simulink model "truck_turn_pid"  (R2024a)
settings: Solver=VariableStepAuto  StartTime=0.0  StopTime=1000  RelTol=1e-3
libraries: slpidlib x2, truck_lib x2
settings Model: Creator=adriaeik  LastModifiedBy=eikel

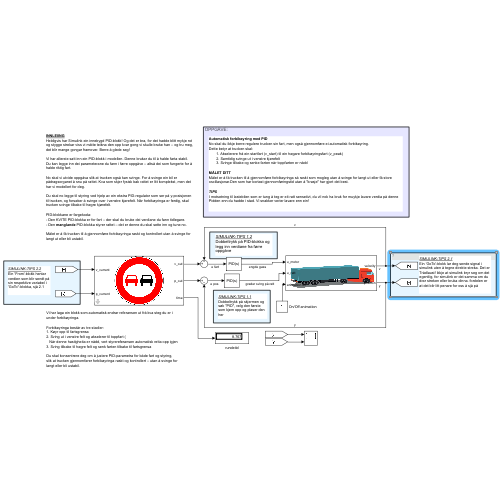
[thumbnail: Simulink's stored preview of the top-level diagram]
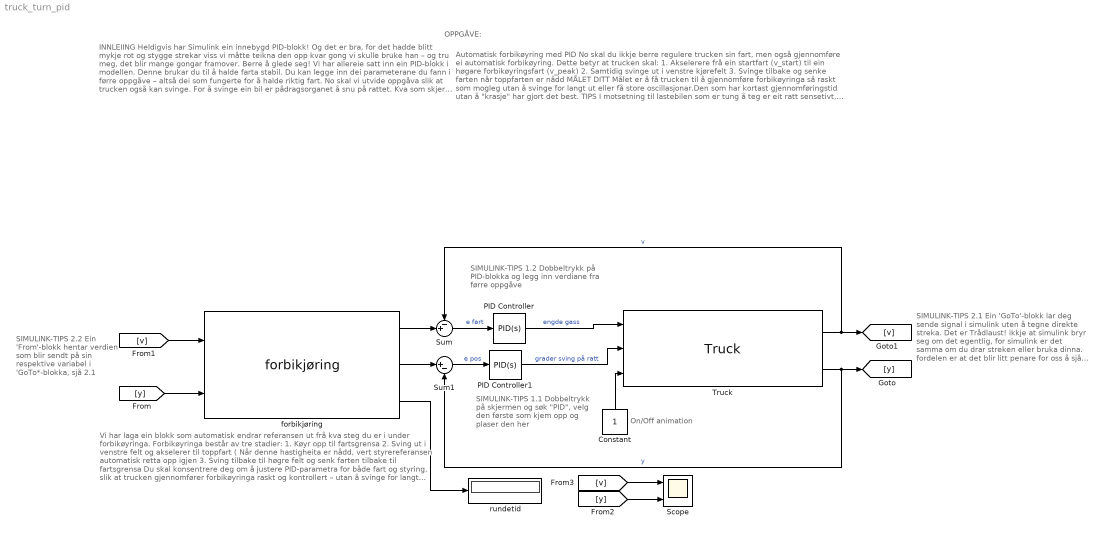
== system truck_turn_pid ==
  note: SIMULINK-TIPS 1.2
      | Dobbeltrykk på PID-blokka og legg inn verdiane fra førre oppgåve
  note: On/Off animation
  note: SIMULINK-TIPS 1.1
      | Dobbeltrykk på skjermen og søk "PID", velg den første som kjem opp og plaser den her
  note: SIMULINK-TIPS 2.1
      | Ein 'GoTo'-blokk lar deg sende signal i simulink uten å tegne direkte streka. Det er Trådlaust! ikkje at simulink bryr seg om det egentlig, for simulink er det samma om du drar streken eller bruka dinna. fordelen er at det blir litt penare for oss å sjå på
  note: INNLEIING
      | Heldigvis har Simulink ein innebygd PID-blokk! Og det er bra, for det hadde blitt mykje rot og stygge strekar viss vi måtte teikna den opp kvar gong vi skulle bruke han – og tru meg, det blir mange gongar framover. Berre å glede seg!
      |
      | Vi har allereie satt inn ein PID-blokk i modellen. Denne brukar du til å halde farta stabil. Du kan legge inn dei parameterane du fann i førre oppgåve – altså dei som fungerte for å halde riktig fart.
      |
      | No skal vi utvide oppgåva slik at trucken også kan svinge. For å svinge ein bil er pådragsorganet å snu på rattet. Kva som skjer fysisk bak rattet er litt komplekst, men det har vi modellert for deg.
      |
      | Du skal no legge til styring ved hjelp av ein ekstra PID-regulator som ser på y-posisjonen til trucken, og forsøker å svinge over i venstre kjørefelt. Når forbikøyringa er ferdig, skal trucken svinge tilbake til høgre kjørefelt.
      |
      | PID-blokkane er fargekoda:
      | - Den KVITE PID-blokka er for fart – der skal du bruke dei verdiane du fann tidlegare.
      | - Den manglande PID-blokka styrer rattet – det er denne du skal sette inn og tune no.
      |
      | Målet er å få trucken til å gjennomføre forbikøyringa raskt og kontrollert utan å svinge for langt ut eller bli ustabil.
  note: OPPGÅVE:
  note: Vi har laga ein blokk som automatisk endrar referansen ut frå kva steg du er i under forbikøyringa.
      |
      | Forbikøyringa består av tre stadier:
      | 1. Køyr opp til fartsgrensa
      | 2. Sving ut i venstre felt og akselerer til toppfart (
      | Når denne hastigheita er nådd, vert styrereferansen automatisk retta opp igjen
      | 3. Sving tilbake til høgre felt og senk farten tilbake til fartsgrensa
      |
      | Du skal konsentrere deg om å justere PID-parametra for både fart og styring,
      | slik at trucken gjennomfører forbikøyringa raskt og kontrollert – utan å svinge for langt eller bli ustabil.
  note: Automatisk forbikøyring med PID
      | No skal du ikkje berre regulere trucken sin fart, men også gjennomføre ei automatisk forbikøyring.
      | Dette betyr at trucken skal:
      | 1. Akselerere frå ein startfart (v_start) til ein høgare forbikøyringsfart (v_peak)
      | 2. Samtidig svinge ut i venstre kjørefelt
      | 3. Svinge tilbake og senke farten når toppfarten er nådd
      |
      | MÅLET DITT
      | Målet er å få trucken til å gjennomføre forbikøyringa så raskt som mogleg utan å svinge for langt ut eller få store oscillasjonar.Den som har kortast gjennomføringstid utan å "krasje" har gjort det best.
      |
      | TIPS
      | I motsetning til lastebilen som er tung å teg er eit ratt sensetivt, du vil nok ha bruk for muykje lavare verdia på denne Pidden enn du hadde i stad. Vi snakker verier lavare enn ein!
  note: SIMULINK-TIPS 2.2
      | Ein 'From'-blokk hentar verdien som blir sendt på sin respektive variabel i 'GoTo*-blokka, sjå 2.1
  Constant : Constant
  PID Controller : slpidlib/PID Controller  Controller=PID  Form=Parallel  TimeDomain=Continuous-time  UseExternalTs=off  SampleTime=-1  IntegratorMethod=Forward Euler  FilterMethod=Forward Euler  ControllerParametersSource=internal  P=1500000  I=9  UseKiTs=off  D=100  UseExternalDerivativeSource=off  N=100  UseFilter=on  TunerSelectOption=Transfer Function Based (PID Tuner App)  InitialConditionSource=internal  InitialConditionForIntegrator=0  InitialConditionForFilter=0  DifferentiatorICPrevScaledInput=0  ExternalReset=none  TrackingMode=off  Kt=1  LimitOutput=off  SatLimitsSource=internal  UpperSaturationLimit=inf  LowerSaturationLimit=-inf  LinearizeAsGain=on  AntiWindupMode=none  Kb=1  LimitIntegrator=off  UpperIntegratorSaturationLimit=inf  LowerIntegratorSaturationLimit=-inf  POutMin=[]  POutMax=[]  IOutMin=[]  IOutMax=[]  DOutMin=[]  DOutMax=[]  NOutMin=[]  NOutMax=[]  SumOutMin=[]  SumOutMax=[]  SaturationOutMin=[]  SaturationOutMax=[]  PParamMin=[]  PParamMax=[]  IParamMin=[]  IParamMax=[]  DParamMin=[]  DParamMax=[]  NParamMin=[]  NParamMax=[]  KbParamMin=[]  KbParamMax=[]  KtParamMin=[]  KtParamMax=[]  KbOutMin=[]  KbOutMax=[]  KtOutMin=[]  KtOutMax=[]  IntegratorOutMin=[]  IntegratorOutMax=[]  FilterOutMin=[]  FilterOutMax=[]  SumI1OutMin=[]  SumI1OutMax=[]  SumI2OutMin=[]  SumI2OutMax=[]  SumI3OutMin=[]  SumI3OutMax=[]  SumI4OutMin=[]  SumI4OutMax=[]  SumDOutMin=[]  SumDOutMax=[]  DifferentiatorOutMin=[]  DifferentiatorOutMax=[]  FilterDiffOutCoefMin=[]  FilterDiffOutCoefMax=[]  ReciprocalOutMin=[]  ReciprocalOutMax=[]  SumDenOutMin=[]  SumDenOutMax=[]  SumNumOutMin=[]  SumNumOutMax=[]  DivideOutMin=[]  DivideOutMax=[]  UdiffTsProdOutMin=[]  UdiffTsProdOutMax=[]  NTsProdOutMin=[]  NTsProdOutMax=[]  UintegralTsProdOutMin=[]  UintegralTsProdOutMax=[]  UngainTsProdOutMin=[]  UngainTsProdOutMax=[]  ClampingZeroOutDataTypeStr=Inherit: Inherit via back propagation  ClampingZeroOutMin=[]  ClampingZeroOutMax=[]  FilterDenConstantOutDataTypeStr=Inherit: Inherit via back propagation  FilterDenConstantOutMin=[]  FilterDenConstantOutMax=[]  PCopyOutDataTypeStr=Inherit: Inherit via back propagation  PCopyOutMin=[]  PCopyOutMax=[]  NCopyOutDataTypeStr=Inherit: Inherit via back propagation  NCopyOutMin=[]  NCopyOutMax=[]  IntegratorContinuousStateAttributes=''  IntegratorStateMustResolveToSignalObject=off  IntegratorRTWStateStorageClass=Auto  FilterContinuousStateAttributes=''  FilterStateMustResolveToSignalObject=off  FilterRTWStateStorageClass=Auto  ParallelPVariant=InternalParameters  IdealPVariant=Disabled  IVariant=InternalParameters  DVariant=InternalParameters  IntegratorVariant=Continuous  SatVariant=Disabled  AWVariant=Passthrough  PCopyVariant=Disabled  TRVariant=Disabled  FdbkBlocksVariant=Forward  IdealPFdbkVariant=Disabled  SatFdbkVariant=Disabled  DerivativeFilterVariant=ContFilter  NVariant=InternalParameters  NCopyVariant=Disabled  FilterICVariant=InternalICsFilter  IntegratorICVariant=InternalICs  ExternalResetVariant=Disabled  TRSumVariant=Passthrough  SumFdbkVariant=Disabled  SumVariant=Sum_PID  TsampFilterVariant=InternalTs  TsampNgainVariant=Passthrough  TsampIntegralVariant=Disabled_SignalSpec  ExternalSaturationOutDataTypeStr=Inherit: Same as second input  DerivativeSourceVariant=ErrorSignal
  PID Controller1 : slpidlib/PID Controller  Controller=PID  Form=Parallel  TimeDomain=Continuous-time  UseExternalTs=off  SampleTime=-1  IntegratorMethod=Forward Euler  FilterMethod=Forward Euler  ControllerParametersSource=internal  P=0.05  I=10  UseKiTs=on  D=10  UseExternalDerivativeSource=off  N=100  UseFilter=on  TunerSelectOption=Transfer Function Based (PID Tuner App)  InitialConditionSource=internal  InitialConditionForIntegrator=0  InitialConditionForFilter=0  DifferentiatorICPrevScaledInput=0  ExternalReset=none  TrackingMode=off  Kt=1  LimitOutput=off  SatLimitsSource=internal  UpperSaturationLimit=inf  LowerSaturationLimit=-inf  LinearizeAsGain=on  AntiWindupMode=none  Kb=1  LimitIntegrator=off  UpperIntegratorSaturationLimit=inf  LowerIntegratorSaturationLimit=-inf  POutMin=[]  POutMax=[]  IOutMin=[]  IOutMax=[]  DOutMin=[]  DOutMax=[]  NOutMin=[]  NOutMax=[]  SumOutMin=[]  SumOutMax=[]  SaturationOutMin=[]  SaturationOutMax=[]  PParamMin=[]  PParamMax=[]  IParamMin=[]  IParamMax=[]  DParamMin=[]  DParamMax=[]  NParamMin=[]  NParamMax=[]  KbParamMin=[]  KbParamMax=[]  KtParamMin=[]  KtParamMax=[]  KbOutMin=[]  KbOutMax=[]  KtOutMin=[]  KtOutMax=[]  IntegratorOutMin=[]  IntegratorOutMax=[]  FilterOutMin=[]  FilterOutMax=[]  SumI1OutMin=[]  SumI1OutMax=[]  SumI2OutMin=[]  SumI2OutMax=[]  SumI3OutMin=[]  SumI3OutMax=[]  SumI4OutMin=[]  SumI4OutMax=[]  SumDOutMin=[]  SumDOutMax=[]  DifferentiatorOutMin=[]  DifferentiatorOutMax=[]  FilterDiffOutCoefMin=[]  FilterDiffOutCoefMax=[]  ReciprocalOutMin=[]  ReciprocalOutMax=[]  SumDenOutMin=[]  SumDenOutMax=[]  SumNumOutMin=[]  SumNumOutMax=[]  DivideOutMin=[]  DivideOutMax=[]  UdiffTsProdOutMin=[]  UdiffTsProdOutMax=[]  NTsProdOutMin=[]  NTsProdOutMax=[]  UintegralTsProdOutMin=[]  UintegralTsProdOutMax=[]  UngainTsProdOutMin=[]  UngainTsProdOutMax=[]  ClampingZeroOutDataTypeStr=Inherit: Inherit via back propagation  ClampingZeroOutMin=[]  ClampingZeroOutMax=[]  FilterDenConstantOutDataTypeStr=Inherit: Inherit via back propagation  FilterDenConstantOutMin=[]  FilterDenConstantOutMax=[]  PCopyOutDataTypeStr=Inherit: Inherit via back propagation  PCopyOutMin=[]  PCopyOutMax=[]  NCopyOutDataTypeStr=Inherit: Inherit via back propagation  NCopyOutMin=[]  NCopyOutMax=[]  IntegratorContinuousStateAttributes=''  IntegratorStateMustResolveToSignalObject=off  IntegratorRTWStateStorageClass=Auto  FilterContinuousStateAttributes=''  FilterStateMustResolveToSignalObject=off  FilterRTWStateStorageClass=Auto  ParallelPVariant=InternalParameters  IdealPVariant=Disabled  IVariant=InternalParameters  DVariant=InternalParameters  IntegratorVariant=Continuous  SatVariant=Disabled  AWVariant=Passthrough  PCopyVariant=Disabled  TRVariant=Disabled  FdbkBlocksVariant=Forward  IdealPFdbkVariant=Disabled  SatFdbkVariant=Disabled  DerivativeFilterVariant=ContFilter  NVariant=InternalParameters  NCopyVariant=Disabled  FilterICVariant=InternalICsFilter  IntegratorICVariant=InternalICs  ExternalResetVariant=Disabled  TRSumVariant=Passthrough  SumFdbkVariant=Disabled  SumVariant=Sum_PID  TsampFilterVariant=InternalTs  TsampNgainVariant=Passthrough  TsampIntegralVariant=Disabled_SignalSpec  ExternalSaturationOutDataTypeStr=Inherit: Same as second input  DerivativeSourceVariant=ErrorSignal
  Scope : Scope  NumInputPorts=2
  Sum : Sum  Inputs=-+|
  Sum1 : Sum  Inputs=|+-
  Truck : truck_lib/Truck  SystemSampleTime=-1  VariantActivationTime=update diagram  AllowFlexibleInterface=on  Latency=0  AutoFrameSizeCalculation=off
      link override C_psi: P=1
  forbikjøring : truck_lib/forbikjøring  speedlimit=10  wrooooom=20
  rundetid : Display
  wires:
  Truck/1 -> [v], Sum/1  "v"
  forbikjøring/1 -> Sum/2
  Sum/1 -> PID Controller/1  "e fart"
  PID Controller/1 -> Truck/1  "engde gass"
  forbikjøring/3 -> rundetid/1
  PID Controller1/1 -> Truck/2  "grader sving på ratt"
  forbikjøring/2 -> Sum1/1
  Truck/2 -> Sum1/2, [y]  "y"
  Sum1/1 -> PID Controller1/1  "e pos"
  [y] -> forbikjøring/2
  [v] -> forbikjøring/1
  [v] -> Scope/1
  [y] -> Scope/2
  Constant/1 -> Truck/3
